simulink model "inner_pd_discrete_test"  (R2016a)
settings: Solver=VariableStepAuto  StartTime=0.0  StopTime=60  RelTol=1e-3
values from neighbouring files (symbols this model uses):
  max_ang_ref = pi/8    (= 0.392699081699)    [init.m]
undefined symbols (not defined in the file or in its folder): inner_h, k, omega_max_lim, omega_min_lim
settings Model: Creator=Daniel  LastModifiedBy=mgreiff
settings DataIOCC: LimitDataPoints=on
settings DebuggingCC: AllowSymbolicDim=off
settings ModelReferenceCC: PropagateSignalLabelsOutOfModel=off
settings GRTTargetCC: GeneratePreprocessorConditionals=Use local settings

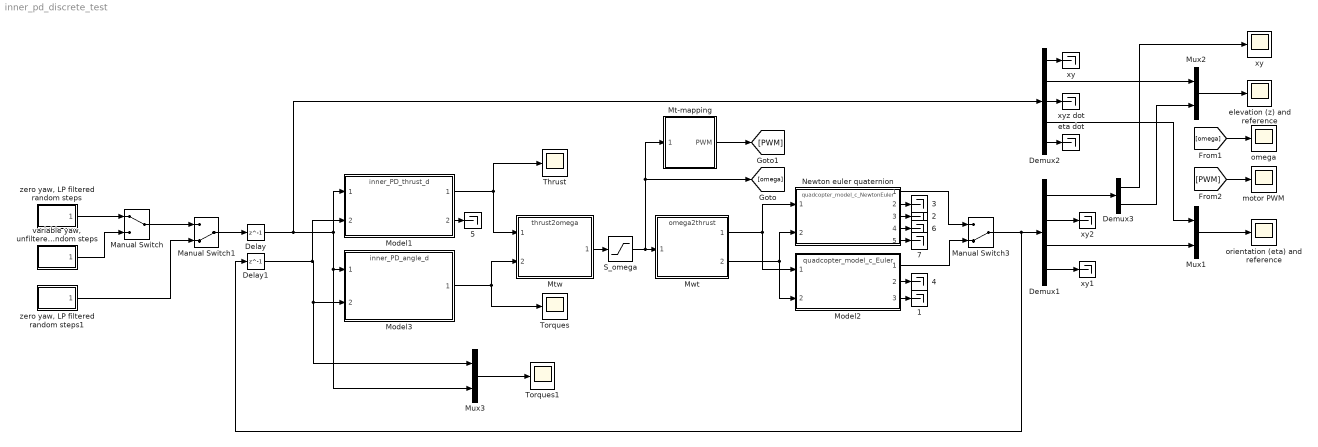
== system inner_pd_discrete_test ==
     {1..7} (7 alike) : Terminator
  "   eta dot" : Terminator
  "   xy" : Terminator
  "   xy1" : Terminator
  "   xy2" : Terminator
  "  xyz dot" : Terminator
  Delay : Delay  DelayLength=1  InitialCondition=0  SampleTime=inner_h
  Delay1 : Delay  DelayLength=1  InitialCondition=0  SampleTime=inner_h
  Demux1 : Demux  Outputs=[3,3,3,3]
  Demux2 : Demux  Outputs=[2,1,3,3,3]
  Demux3 : Demux  Outputs=[2,1]
  Manual Switch : ManualSwitch
  Manual Switch1 : ManualSwitch  CurrentSetting=0
  Manual Switch3 : ManualSwitch  CurrentSetting=0
  Model1 : ModelReference  ModelNameDialog=inner_PD_thrust_d.slx  SimulationMode=Normal  ModelReferenceVersion=1.81
  Model2 : ModelReference  ModelNameDialog=quadcopter_model_c_Euler.mdl  SimulationMode=Normal  ModelReferenceVersion=1.167
  Model3 : ModelReference  ModelNameDialog=inner_PD_angle_d.slx  SimulationMode=Normal  ModelReferenceVersion=1.85
  Mt-mapping : Subsystem
  Mtw : ModelReference  ModelNameDialog=thrust2omega.mdl  SimulationMode=Normal  ModelReferenceVersion=1.3
  Mux1 : Mux  Inputs=2
  Mux2 : Mux  Inputs=2
  Mux3 : Mux  Inputs=2
  Mwt : ModelReference  ModelNameDialog=omega2thrust.mdl  SimulationMode=Normal  ModelReferenceVersion=1.3
  Newton euler quaternion : ModelReference  ModelNameDialog=quadcopter_model_c_NewtonEuler.mdl  SimulationMode=Normal  ModelReferenceVersion=1.325
  S_omega : Saturate  UpperLimit=omega_max_lim  LowerLimit=omega_min_lim
  Thrust : Scope
  Torques : Scope
  Torques1 : Scope
  elevation (z) and reference : Scope
  motor PWM : Scope
  "omega " : Scope
  orientation (eta) and reference : Scope
  "variable yaw, unfiltered random steps" : Subsystem
  xy : Scope
  "zero yaw, LP filtered random steps" : Subsystem
  "zero yaw, LP filtered random steps1" : Subsystem
  wires:
  "variable yaw, unfiltered random steps"/1(reference) -> Manual Switch/2
  "zero yaw, LP filtered random steps"/1(reference) -> Manual Switch/1
  Mux2/1 -> elevation (z) and reference/1
  Manual Switch3/1 -> Delay1/1, Demux1/1
  Mux1/1 -> orientation (eta) and reference/1
  Demux2/3 -> "  xyz dot"/1
  Demux2/5 -> "   eta dot"/1
  Demux2/1 -> "   xy"/1
  Demux1/1 -> Demux3/1
  [omega] -> "omega "/1
  Delay/1 -> Demux2/1, Mux3/2, Model3/1, Model1/1
  Delay1/1 -> Model1/2, Mux3/1, Model3/2
  Demux1/4 -> "   xy1"/1
  Demux1/2 -> "   xy2"/1
  Demux3/1 -> xy/1
  Mt-mapping/1(PWM) -> [PWM]
  [PWM] -> motor PWM/1
  Manual Switch/1 -> Manual Switch1/1
  Manual Switch1/1 -> Delay/1
  "zero yaw, LP filtered random steps1"/1(reference) -> Manual Switch1/2
  Model2/3 -> "   1"/1
  Newton euler quaternion/3 -> "   2"/1
  Newton euler quaternion/2 -> "   3"/1
  Model2/2 -> "   4"/1
  Model2/1 -> Manual Switch3/2
  Newton euler quaternion/1 -> Manual Switch3/1
  Mtw/1 -> S_omega/1
  Mwt/1 -> Model2/1, Newton euler quaternion/1
  Mwt/2 -> Model2/2, Newton euler quaternion/2
  S_omega/1 -> [omega], Mt-mapping/1(omega), Mwt/1
  Model3/1 -> Torques/1, Mtw/2
  Model1/1 -> Thrust/1, Mtw/1
  Model1/2 -> "   5"/1
  Mux3/1 -> Torques1/1
  Newton euler quaternion/4 -> "   6"/1
  Newton euler quaternion/5 -> "   7"/1
  Demux2/2 -> Mux2/1
  Demux3/2 -> Mux2/2
  Demux1/3 -> Mux1/2
  Demux2/4 -> Mux1/1

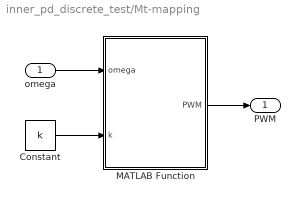
== system inner_pd_discrete_test/Mt-mapping ==
  omega : Inport
  Constant : Constant  Value=k
  MATLAB Function : MATLAB Function  TreatAsAtomicUnit=on
  PWM : Outport
  wires:
  MATLAB Function/1(PWM) -> PWM/1
  omega/1 -> MATLAB Function/1(omega)
  Constant/1 -> MATLAB Function/2(k)

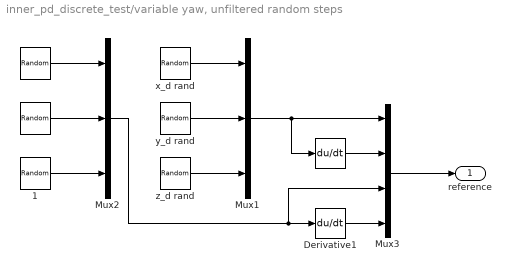
== system inner_pd_discrete_test/variable yaw, unfiltered random steps ==
  " " : UniformRandomNumber  Minimum=-0.8  Maximum=0.8  Seed=4  SampleTime=10
  "   " : UniformRandomNumber  Minimum=-0.2  Maximum=0.2  Seed=3  SampleTime=10
  "        " : Derivative
  " 1" : UniformRandomNumber  Minimum=-0.8  Maximum=0.8  Seed=5  SampleTime=10
  Derivative1 : Derivative
  Mux1 : Mux  Inputs=3
  Mux2 : Mux  Inputs=3
  Mux3 : Mux  Inputs=[3,3,3,3]
  x_d rand : UniformRandomNumber  Minimum=-30  Maximum=30  SampleTime=10
  y_d rand : UniformRandomNumber  Minimum=-30  Maximum=30  Seed=1  SampleTime=10
  z_d rand : UniformRandomNumber  Minimum=0  Maximum=15  Seed=2  SampleTime=10
  reference : Outport
  wires:
  Mux1/1 -> "        "/1, Mux3/1
  Mux3/1 -> reference/1
  Derivative1/1 -> Mux3/4
  "        "/1 -> Mux3/2
  Mux2/1 -> Mux3/3, Derivative1/1
  "   "/1 -> Mux2/1
  " "/1 -> Mux2/2
  " 1"/1 -> Mux2/3
  x_d rand/1 -> Mux1/1
  y_d rand/1 -> Mux1/2
  z_d rand/1 -> Mux1/3

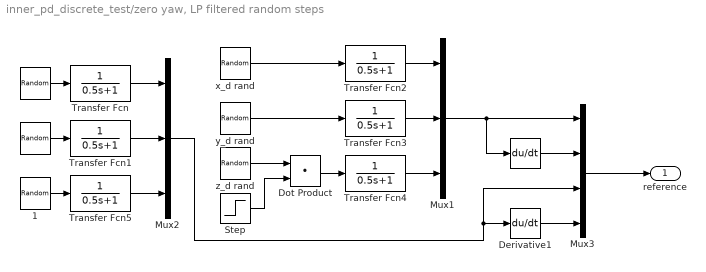
== system inner_pd_discrete_test/zero yaw, LP filtered random steps ==
  " " : UniformRandomNumber  Minimum=-max_ang_ref  Maximum=max_ang_ref  Seed=4  SampleTime=10
  "   " : UniformRandomNumber  Minimum=-max_ang_ref  Maximum=max_ang_ref  Seed=3  SampleTime=10
  "        " : Derivative
  " 1" : UniformRandomNumber  Minimum=-max_ang_ref  Maximum=max_ang_ref  Seed=5  SampleTime=10
  Derivative1 : Derivative
  Dot Product : DotProduct  InputSameDT=on  OutDataTypeStr=Inherit: Inherit via internal rule
  Mux1 : Mux  Inputs=3
  Mux2 : Mux  Inputs=3
  Mux3 : Mux  Inputs=[3,3,3,3]
  Step : Step  Time=40  Before=1  After=0  SampleTime=0
  Transfer Fcn{,1..5} (6 alike) : TransferFcn  Denominator=[0.5 1]
  x_d rand : UniformRandomNumber  Minimum=-30  Maximum=30  SampleTime=10
  y_d rand : UniformRandomNumber  Minimum=-30  Maximum=30  Seed=1  SampleTime=10
  z_d rand : UniformRandomNumber  Minimum=0  Maximum=3  Seed=2  SampleTime=10
  reference : Outport
  wires:
  Mux1/1 -> "        "/1, Mux3/1
  Mux3/1 -> reference/1
  Derivative1/1 -> Mux3/4
  "        "/1 -> Mux3/2
  Mux2/1 -> Mux3/3, Derivative1/1
  "   "/1 -> Transfer Fcn/1
  " "/1 -> Transfer Fcn1/1
  Transfer Fcn/1 -> Mux2/1
  Transfer Fcn1/1 -> Mux2/2
  Transfer Fcn5/1 -> Mux2/3
  x_d rand/1 -> Transfer Fcn2/1
  y_d rand/1 -> Transfer Fcn3/1
  Transfer Fcn2/1 -> Mux1/1
  Transfer Fcn3/1 -> Mux1/2
  Transfer Fcn4/1 -> Mux1/3
  Step/1 -> Dot Product/2
  z_d rand/1 -> Dot Product/1
  Dot Product/1 -> Transfer Fcn4/1
  " 1"/1 -> Transfer Fcn5/1

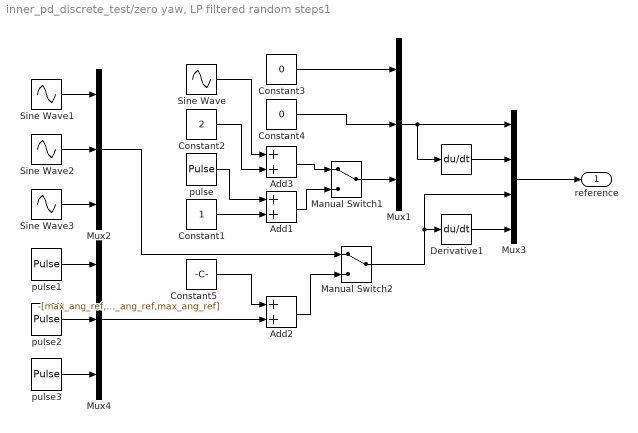
== system inner_pd_discrete_test/zero yaw, LP filtered random steps1 ==
  "        " : Derivative
  Add1 : Sum
  Add2 : Sum
  Add3 : Sum
  Constant1 : Constant
  Constant2 : Constant  Value=2
  Constant3 : Constant  Value=0
  Constant4 : Constant  Value=0
  Constant5 : Constant  Value=-[max_ang_ref,max_ang_ref,max_ang_ref]
  Derivative1 : Derivative
  Manual Switch1 : ManualSwitch
  Manual Switch2 : ManualSwitch
  Mux1 : Mux  Inputs=3
  Mux2 : Mux  Inputs=3
  Mux3 : Mux  Inputs=[3,3,3,3]
  Mux4 : Mux  Inputs=3
  Sine Wave : Sin  SampleTime=0
  Sine Wave1 : Sin  Amplitude=max_ang_ref  SampleTime=0
  Sine Wave2 : Sin  Amplitude=max_ang_ref  Phase=pi/2
  Sine Wave3 : Sin  Amplitude=max_ang_ref  Phase=pi  SampleTime=0
  pulse : DiscretePulseGenerator  PulseType=Time based  Amplitude=2  Period=10  PulseWidth=50
  pulse1 : DiscretePulseGenerator  PulseType=Time based  Amplitude=max_ang_ref*2  Period=10  PulseWidth=50
  pulse2 : DiscretePulseGenerator  PulseType=Time based  Amplitude=max_ang_ref*2  Period=10  PulseWidth=50
  pulse3 : DiscretePulseGenerator  PulseType=Time based  Amplitude=max_ang_ref*2  Period=10  PulseWidth=50
  reference : Outport
  wires:
  Mux1/1 -> "        "/1, Mux3/1
  Mux3/1 -> reference/1
  Derivative1/1 -> Mux3/4
  "        "/1 -> Mux3/2
  Sine Wave1/1 -> Mux2/1
  Sine Wave2/1 -> Mux2/2
  Sine Wave3/1 -> Mux2/3
  Constant3/1 -> Mux1/1
  Constant4/1 -> Mux1/2
  Sine Wave/1 -> Add3/1
  Constant2/1 -> Add3/2
  Add3/1 -> Manual Switch1/1
  Manual Switch1/1 -> Mux1/3
  Add1/1 -> Manual Switch1/2
  Constant1/1 -> Add1/2
  pulse/1 -> Add1/1
  pulse1/1 -> Mux4/1
  pulse2/1 -> Mux4/2
  pulse3/1 -> Mux4/3
  Constant5/1 -> Add2/1
  Mux4/1 -> Add2/2
  Mux2/1 -> Manual Switch2/1
  Add2/1 -> Manual Switch2/2
  Manual Switch2/1 -> Mux3/3, Derivative1/1

== matlab function inner_pd_discrete_test/Mt-mapping/MATLAB Function ==
  data: omega input; PWM output; k input
function PWM = Mt(omega, k)
%#codegen
rotor_thrusts = k.*omega.^2;
beta1 = 0.0877;
beta2 = 0.0660;
PWM =  -beta1/(2*beta2) + sqrt((beta1/(2*beta2))^2 + rotor_thrusts/beta2);
